simulink model "model"  (R2021a)
settings: Solver=VariableStepAuto  StartTime=0.0  StopTime=10.0  RelTol=1e-3
settings Model: Creator=zlioo  LastModifiedBy=zlioo

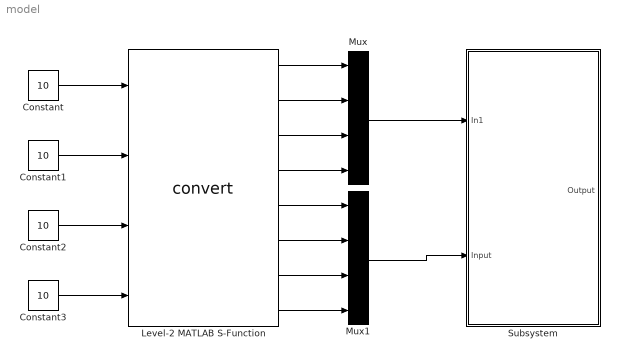
== system model ==
  Constant{,1..3} (4 alike) : Constant  Value=10
  Level-2 MATLAB S-Function : M-S-Function  FunctionName=convert
  Mux : Mux
  Mux1 : Mux
  Subsystem : Subsystem
  wires:
  Constant3/1 -> Level-2 MATLAB S-Function/4
  Constant2/1 -> Level-2 MATLAB S-Function/3
  Constant1/1 -> Level-2 MATLAB S-Function/2
  Constant/1 -> Level-2 MATLAB S-Function/1
  Level-2 MATLAB S-Function/1 -> Mux/1
  Level-2 MATLAB S-Function/2 -> Mux/2
  Level-2 MATLAB S-Function/3 -> Mux/3
  Level-2 MATLAB S-Function/4 -> Mux/4
  Level-2 MATLAB S-Function/5 -> Mux1/1
  Level-2 MATLAB S-Function/6 -> Mux1/2
  Level-2 MATLAB S-Function/7 -> Mux1/3
  Level-2 MATLAB S-Function/8 -> Mux1/4
  Mux1/1 -> Subsystem/2(Input)
  Mux/1 -> Subsystem/1(In1)

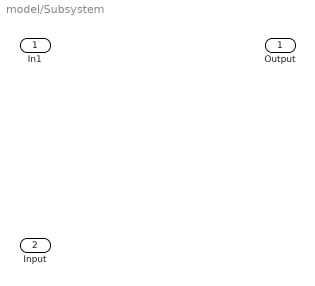
== system model/Subsystem ==
  In1 : Inport
  Input : Inport  Port=2
  Output : Outport
